simulink model "lab6"  (R2021b)
settings: Solver=FixedStepAuto  StartTime=0.0  StopTime=inf  FixedStep=t_s  RelTol=1e-3
undefined symbols (not defined in the file): Amp, angle_target, Bias, Freq, Phase, t_s
libraries: instrumentseriallib x6, slpidlib x2
settings Model: Creator=16970  LastModifiedBy=16970

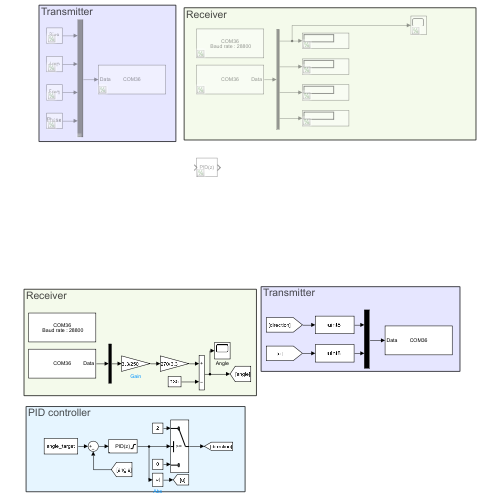
[thumbnail: Simulink's stored preview of the top-level diagram]
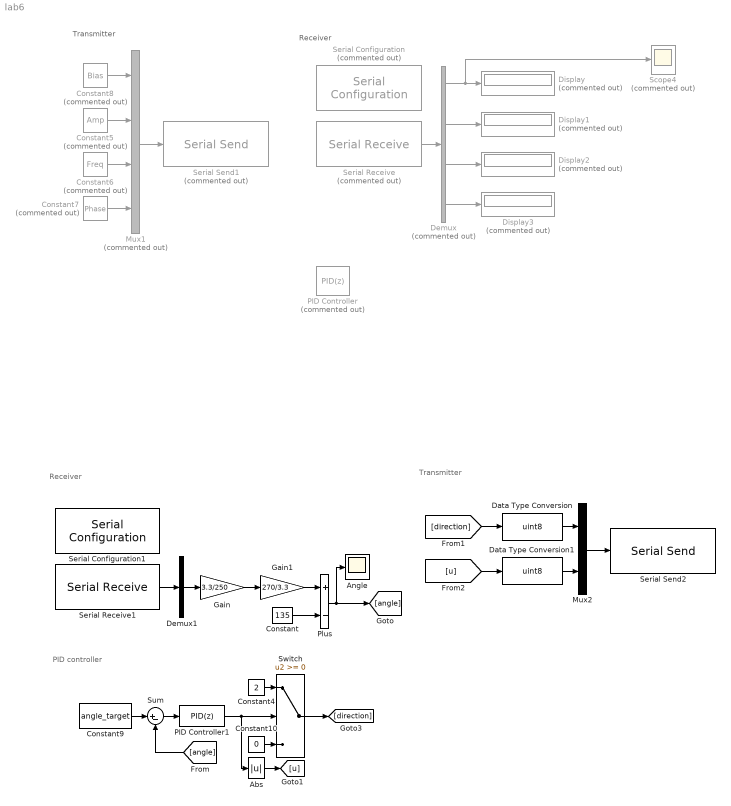
== system lab6 ==
  note: PID controller
  note: Receiver
  note: Transmitter
  note: Transmitter
  note: Receiver
  Abs : Abs
  Angle : Scope
  Constant : Constant  Value=135
  Constant10 : Constant  Value=0
  Constant4 : Constant  Value=2
  Constant5 : Constant  Commented=on  Value=Amp  OutDataTypeStr=uint8  SampleTime=t_s
  Constant6 : Constant  Commented=on  Value=Freq  OutDataTypeStr=uint8  SampleTime=t_s
  Constant7 : Constant  Commented=on  Value=Phase  OutDataTypeStr=uint8  SampleTime=t_s
  Constant8 : Constant  Commented=on  Value=Bias  OutDataTypeStr=uint8  SampleTime=t_s
  Constant9 : Constant  Value=angle_target
  Data Type Conversion : DataTypeConversion  OutDataTypeStr=uint8
  Data Type Conversion1 : DataTypeConversion  OutDataTypeStr=uint8
  Demux : Demux  Commented=on
  Demux1 : Demux  Outputs=1
  Display{,1..3} (4 alike) : Display  Commented=on
  Gain : Gain  Gain=3.3/250
  Gain1 : Gain  Gain=270/3.3
  Mux1 : Mux  Commented=on
  Mux2 : Mux  Inputs=2
  PID Controller : slpidlib/PID Controller  Commented=on  Controller=PID  Form=Parallel  TimeDomain=Discrete-time  UseExternalTs=off  SampleTime=-1  IntegratorMethod=Forward Euler  FilterMethod=Forward Euler  ControllerParametersSource=internal  P=1  I=1  D=0  UseFilter=on  N=100  TunerSelectOption=Transfer Function Based (PID Tuner App)  InitialConditionSource=internal  InitialConditionForIntegrator=0  InitialConditionForFilter=0  DifferentiatorICPrevScaledInput=0  ExternalReset=none  TrackingMode=off  Kt=1  LimitOutput=off  SatLimitsSource=internal  UpperSaturationLimit=inf  LowerSaturationLimit=-inf  LinearizeAsGain=on  AntiWindupMode=none  Kb=1  POutMin=[]  POutMax=[]  IOutMin=[]  IOutMax=[]  DOutMin=[]  DOutMax=[]  NOutMin=[]  NOutMax=[]  SumOutMin=[]  SumOutMax=[]  SaturationOutMin=[]  SaturationOutMax=[]  PParamMin=[]  PParamMax=[]  IParamMin=[]  IParamMax=[]  DParamMin=[]  DParamMax=[]  NParamMin=[]  NParamMax=[]  KbParamMin=[]  KbParamMax=[]  KtParamMin=[]  KtParamMax=[]  KbOutMin=[]  KbOutMax=[]  KtOutMin=[]  KtOutMax=[]  IntegratorOutMin=[]  IntegratorOutMax=[]  FilterOutMin=[]  FilterOutMax=[]  SumI1OutMin=[]  SumI1OutMax=[]  SumI2OutMin=[]  SumI2OutMax=[]  SumI3OutMin=[]  SumI3OutMax=[]  SumI4OutMin=[]  SumI4OutMax=[]  SumDOutMin=[]  SumDOutMax=[]  DifferentiatorOutMin=[]  DifferentiatorOutMax=[]  FilterDiffOutCoefMin=[]  FilterDiffOutCoefMax=[]  ReciprocalOutMin=[]  ReciprocalOutMax=[]  SumDenOutMin=[]  SumDenOutMax=[]  SumNumOutMin=[]  SumNumOutMax=[]  DivideOutMin=[]  DivideOutMax=[]  UdiffTsProdOutMin=[]  UdiffTsProdOutMax=[]  NTsProdOutMin=[]  NTsProdOutMax=[]  UintegralTsProdOutMin=[]  UintegralTsProdOutMax=[]  UngainTsProdOutMin=[]  UngainTsProdOutMax=[]  IntegratorContinuousStateAttributes=''  IntegratorStateMustResolveToSignalObject=off  IntegratorRTWStateStorageClass=Auto  FilterContinuousStateAttributes=''  FilterStateMustResolveToSignalObject=off  FilterRTWStateStorageClass=Auto  ParallelPVariant=InternalParameters  IdealPVariant=Disabled  IVariant=InternalParameters  DVariant=InternalParameters  IntegratorVariant=Discrete  SatVariant=Disabled  AWVariant=Passthrough  PCopyVariant=Disabled  TRVariant=Disabled  FdbkBlocksVariant=Forward  IdealPFdbkVariant=Disabled  SatFdbkVariant=Disabled  DerivativeFilterVariant=ForwardEulerFilter  NVariant=InternalParameters  NCopyVariant=Disabled  FilterICVariant=InternalICsFilter  IntegratorICVariant=InternalICs  ExternalResetVariant=Disabled  TRSumVariant=Passthrough  SumFdbkVariant=Disabled  SumVariant=Sum_PID  TsampFilterVariant=InternalTs  TsampNgainVariant=Passthrough  TsampIntegralVariant=Passthrough  ExternalSaturationOutDataTypeStr=Inherit: Same as second input
  PID Controller1 : slpidlib/PID Controller  Controller=PID  Form=Parallel  TimeDomain=Discrete-time  UseExternalTs=off  SampleTime=-1  IntegratorMethod=Forward Euler  FilterMethod=Forward Euler  ControllerParametersSource=internal  P=1  I=0.5  D=0  UseFilter=on  N=100  TunerSelectOption=Transfer Function Based (PID Tuner App)  InitialConditionSource=internal  InitialConditionForIntegrator=0  InitialConditionForFilter=0  DifferentiatorICPrevScaledInput=0  ExternalReset=none  TrackingMode=off  Kt=1  LimitOutput=on  SatLimitsSource=internal  UpperSaturationLimit=100  LowerSaturationLimit=-100  LinearizeAsGain=on  AntiWindupMode=none  Kb=1  POutMin=[]  POutMax=[]  IOutMin=[]  IOutMax=[]  DOutMin=[]  DOutMax=[]  NOutMin=[]  NOutMax=[]  SumOutMin=[]  SumOutMax=[]  SaturationOutMin=[]  SaturationOutMax=[]  PParamMin=[]  PParamMax=[]  IParamMin=[]  IParamMax=[]  DParamMin=[]  DParamMax=[]  NParamMin=[]  NParamMax=[]  KbParamMin=[]  KbParamMax=[]  KtParamMin=[]  KtParamMax=[]  KbOutMin=[]  KbOutMax=[]  KtOutMin=[]  KtOutMax=[]  IntegratorOutMin=[]  IntegratorOutMax=[]  FilterOutMin=[]  FilterOutMax=[]  SumI1OutMin=[]  SumI1OutMax=[]  SumI2OutMin=[]  SumI2OutMax=[]  SumI3OutMin=[]  SumI3OutMax=[]  SumI4OutMin=[]  SumI4OutMax=[]  SumDOutMin=[]  SumDOutMax=[]  DifferentiatorOutMin=[]  DifferentiatorOutMax=[]  FilterDiffOutCoefMin=[]  FilterDiffOutCoefMax=[]  ReciprocalOutMin=[]  ReciprocalOutMax=[]  SumDenOutMin=[]  SumDenOutMax=[]  SumNumOutMin=[]  SumNumOutMax=[]  DivideOutMin=[]  DivideOutMax=[]  UdiffTsProdOutMin=[]  UdiffTsProdOutMax=[]  NTsProdOutMin=[]  NTsProdOutMax=[]  UintegralTsProdOutMin=[]  UintegralTsProdOutMax=[]  UngainTsProdOutMin=[]  UngainTsProdOutMax=[]  IntegratorContinuousStateAttributes=''  IntegratorStateMustResolveToSignalObject=off  IntegratorRTWStateStorageClass=Auto  FilterContinuousStateAttributes=''  FilterStateMustResolveToSignalObject=off  FilterRTWStateStorageClass=Auto  ParallelPVariant=InternalParameters  IdealPVariant=Disabled  IVariant=InternalParameters  DVariant=InternalParameters  IntegratorVariant=Discrete  SatVariant=Enabled  AWVariant=Passthrough  PCopyVariant=Disabled  TRVariant=Disabled  FdbkBlocksVariant=Forward  IdealPFdbkVariant=Disabled  SatFdbkVariant=Disabled  DerivativeFilterVariant=ForwardEulerFilter  NVariant=InternalParameters  NCopyVariant=Disabled  FilterICVariant=InternalICsFilter  IntegratorICVariant=InternalICs  ExternalResetVariant=Disabled  TRSumVariant=Passthrough  SumFdbkVariant=Disabled  SumVariant=Sum_PID  TsampFilterVariant=InternalTs  TsampNgainVariant=Passthrough  TsampIntegralVariant=Passthrough  ExternalSaturationOutDataTypeStr=Inherit: Same as second input
  Plus : Sum  Inputs=+-
  Scope4 : Scope  Commented=on
  Serial Configuration : instrumentseriallib/Serial Configuration  Priority=-200000  Commented=on  Port=COM36  ComPort=COM36  BaudRate=28800  DataBits=8  Parity=none  StopBits=1  ByteOrder=little-endian  FlowControl=none  Timeout=1000  SimulateUsing=Interpreted execution  BlockInModel=on
  Serial Configuration1 : instrumentseriallib/Serial Configuration  Priority=-200000  Port=COM36  ComPort=COM36  BaudRate=28800  DataBits=8  Parity=none  StopBits=1  ByteOrder=little-endian  FlowControl=none  Timeout=1000  SimulateUsing=Interpreted execution  BlockInModel=on
  Serial Receive : instrumentseriallib/Serial Receive  Priority=1  Commented=on  Port=COM36  ComPort=COM36  DataType=uint8  SaveDataType=uint8  ToggleHeader=on  Header=['H']  ToggleTerminator=on  Terminator=Custom terminator  CustomTerminator=['T']  ToggleDataSize=on  DataSize=[1 4]  EnableBlockingMode=on  ActionDataUnavailable=Error  ActionWhenDataUnavailable=Error  CustomValue=0  SampleTime=t_s  SimulateUsing=Interpreted execution  BlockInModel=on
  Serial Receive1 : instrumentseriallib/Serial Receive  Priority=1  Port=COM36  ComPort=COM36  DataType=uint8  SaveDataType=uint8  ToggleHeader=on  Header=['H']  ToggleTerminator=on  Terminator=Custom terminator  CustomTerminator=['T']  ToggleDataSize=on  DataSize=[1 1]  EnableBlockingMode=on  ActionDataUnavailable=Error  ActionWhenDataUnavailable=Error  CustomValue=0  SampleTime=t_s  SimulateUsing=Interpreted execution  BlockInModel=on
  Serial Send1 : instrumentseriallib/Serial Send  Priority=1  Commented=on  Port=COM36  ComPort=COM36  Header=[]  Terminator=<none>  CustomTerminator=['T']  EnableBlockingMode=on  SimulateUsing=Interpreted execution  BlockInModel=on
  Serial Send2 : instrumentseriallib/Serial Send  Priority=1  Port=COM36  ComPort=COM36  Header=[]  Terminator=<none>  CustomTerminator=['T']  EnableBlockingMode=on  SimulateUsing=Interpreted execution  BlockInModel=on
  Sum : Sum  Inputs=|+-
  Switch : Switch
  wires:
  Serial Receive/1 -> Demux/1
  Demux/2 -> Display1/1
  Demux/3 -> Display2/1
  Demux/4 -> Display3/1
  Constant5/1 -> Mux1/2
  Constant8/1 -> Mux1/1
  Constant6/1 -> Mux1/3
  Demux/1 -> Scope4/1, Display/1
  Mux1/1 -> Serial Send1/1
  Constant7/1 -> Mux1/4
  Serial Receive1/1 -> Demux1/1
  Demux1/1 -> Gain/1
  Mux2/1 -> Serial Send2/1
  Gain/1 -> Gain1/1
  Gain1/1 -> Plus/1
  Constant/1 -> Plus/2
  Plus/1 -> [angle], Angle/1
  Sum/1 -> PID Controller1/1
  Constant9/1 -> Sum/1
  [angle] -> Sum/2
  PID Controller1/1 -> Abs/1, Switch/2
  Constant4/1 -> Switch/1
  Constant10/1 -> Switch/3
  Switch/1 -> [direction]
  [direction] -> Data Type Conversion/1
  Data Type Conversion/1 -> Mux2/1
  [u] -> Data Type Conversion1/1
  Data Type Conversion1/1 -> Mux2/2
  Abs/1 -> [u]
